simulink model "sm_SG"  (R2019a)
settings: Solver=FixedStepDiscrete  StartTime=0.0  StopTime=stop_time  RelTol=1e-3
InitFcn:
  | sm_callback_init
StopFcn:
  | sm_callback_stop
values from neighbouring files (symbols this model uses):
  mp = sm_init_avalon_signals(mp)    [sm_callback_init.m]
libraries: simulink x3
settings Model: Creator=Ross  LastModifiedBy=Ross
settings DataIOCC: ReturnWorkspaceOutputs=off
settings OptimizationCC: BlockReduction=off  ConditionallyExecuteInputs=off  DefaultParameterBehavior=Inlined
settings DebuggingCC: ReadBeforeWriteMsg=DisableAll  WriteAfterWriteMsg=DisableAll  WriteAfterReadMsg=DisableAll  AlgebraicLoopMsg=error  MultiTaskDSMMsg=none  SingleTaskRateTransMsg=error  PregeneratedLibrarySubsystemCodeDiagnostic=none  ArithmeticOperatorsInVariantConditions=warning
settings HardwareCC: ProdBitPerPointer=32  ProdBitPerSizeT=32  ProdBitPerPtrDiffT=32  ProdLargestAtomicFloat=None  ProdIntDivRoundTo=Undefined  ProdEndianess=Unspecified  ProdWordSize=32  ProdHWDeviceType=ASIC/FPGA->ASIC/FPGA  TargetBitPerPointer=64  TargetBitPerSizeT=64  TargetBitPerPtrDiffT=64  TargetLongLongMode=on  TargetIntDivRoundTo=Zero  TargetEndianess=LittleEndian  TargetWordSize=64  TargetHWDeviceType=Custom Processor->MATLAB Host Computer  ProdEqTarget=off
settings ModelReferenceCC: UpdateModelReferenceTargets=IfOutOfDate
settings SFSimCC: SFSimEcho=off  SimUseLocalCustomCode=off
settings RTWCC: RTWUseLocalCustomCode=off

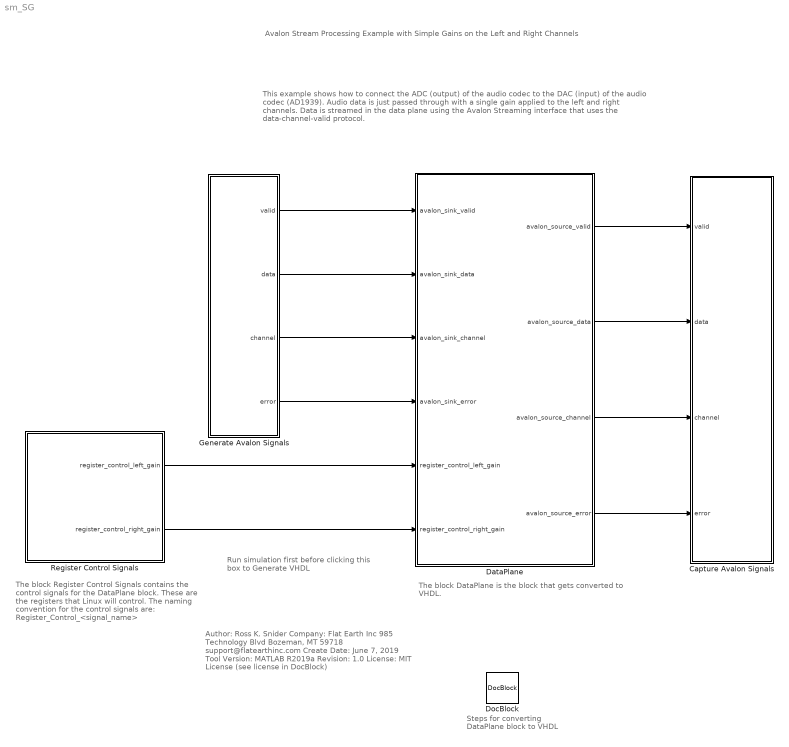
== system sm_SG ==
  note: The block DataPlane is the block that gets converted to VHDL.
  note: Author:          Ross K. Snider
      | Company:     Flat Earth Inc
      |                       985 Technology Blvd
      |                       Bozeman, MT 59718
      |                       support@flatearthinc.com
      | Create Date:  June 7, 2019
      | Tool Version:  MATLAB R2019a
      | Revision:        1.0
      | License:          MIT License (see license in DocBlock)
  note: This example shows how to connect the ADC (output) of the audio codec to the DAC (input) of the audio codec (AD1939). Audio data is just passed through with a single gain applied to the left and right channels. Data is streamed in the data plane using the Avalon Streaming interface that uses the data-channel-valid protocol.
  note: Steps for converting
      | DataPlane block
      | to VHDL
  note: Avalon Stream Processing Example
      | with Simple Gains on the Left and Right Channels
  note: Run simulation first
      | before clicking this box to
      | Generate VHDL
  note: The block Register Control Signals contains
      | the control signals for the DataPlane block.
      | These are the registers that Linux will control.
      | The naming convention for the control
      | signals are:  Register_Control_<signal_name>
  Capture Avalon Signals : Subsystem
  DataPlane : Subsystem  TreatAsAtomicUnit=on
  DocBlock : simulink/Model-Wide Utilities/DocBlock  DocumentType=HTML
  Generate Avalon Signals : Subsystem
  Register Control Signals : Subsystem
  wires:
  Generate Avalon Signals/2(data) -> DataPlane/2(avalon_sink_data)
  Generate Avalon Signals/1(valid) -> DataPlane/1(avalon_sink_valid)
  Generate Avalon Signals/3(channel) -> DataPlane/3(avalon_sink_channel)
  Generate Avalon Signals/4(error) -> DataPlane/4(avalon_sink_error)
  DataPlane/2(avalon_source_data) -> Capture Avalon Signals/2(data)
  DataPlane/1(avalon_source_valid) -> Capture Avalon Signals/1(valid)
  DataPlane/3(avalon_source_channel) -> Capture Avalon Signals/3(channel)
  DataPlane/4(avalon_source_error) -> Capture Avalon Signals/4(error)
  Register Control Signals/1(register_control_left_gain) -> DataPlane/5(register_control_left_gain)
  Register Control Signals/2(register_control_right_gain) -> DataPlane/6(register_control_right_gain)

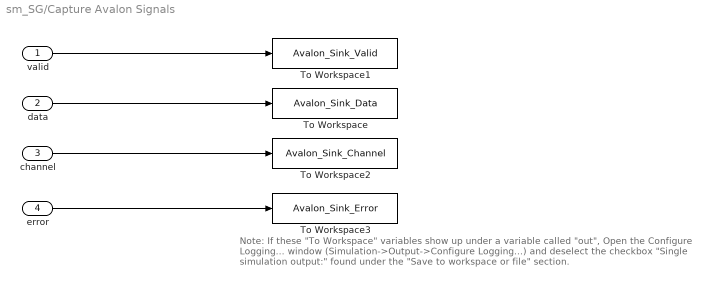
== system sm_SG/Capture Avalon Signals ==
  note: Note:  If these "To Workspace" variables show up under a variable called "out",
      | Open the Configure Logging... window (Simulation->Output->Configure Logging...)
      | and deselect the checkbox "Single simulation output:" found under the "Save to workspace or file" section.
  valid : Inport
  data : Inport  Port=2
  channel : Inport  Port=3
  error : Inport  Port=4
  To Workspace : ToWorkspace  VariableName=Avalon_Sink_Data  SaveFormat=Timeseries  SampleTime=-1
  To Workspace1 : ToWorkspace  VariableName=Avalon_Sink_Valid  SaveFormat=Timeseries  SampleTime=-1
  To Workspace2 : ToWorkspace  VariableName=Avalon_Sink_Channel  SaveFormat=Timeseries  SampleTime=-1
  To Workspace3 : ToWorkspace  VariableName=Avalon_Sink_Error  SaveFormat=Timeseries  SampleTime=-1
  wires:
  data/1 -> To Workspace/1
  valid/1 -> To Workspace1/1
  error/1 -> To Workspace3/1
  channel/1 -> To Workspace2/1

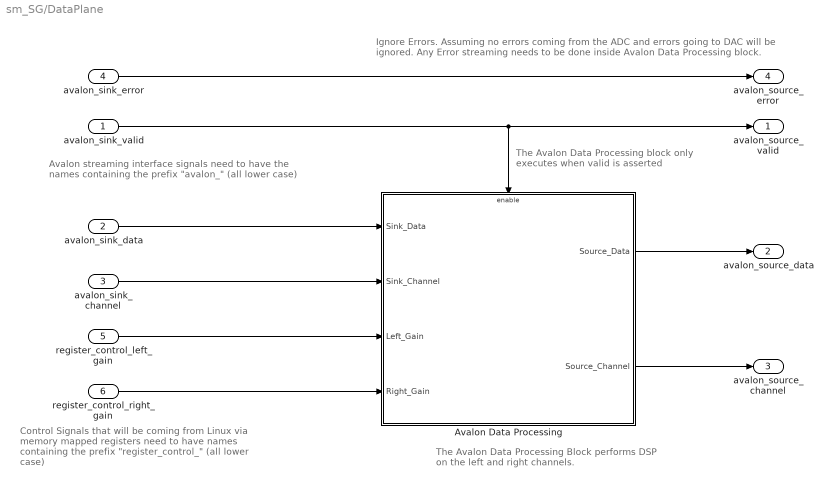
== system sm_SG/DataPlane ==
  note: Control Signals that will be coming from Linux via
      | memory mapped registers need to have names
      | containing the prefix "register_control_"
      | (all lower case)
  note: The Avalon Data Processing Block
      | performs DSP on the left and right channels.
  note: The Avalon Data Processing block
      | only executes when valid is asserted
  note: Ignore Errors.
      | Assuming no errors coming from the ADC and errors going to DAC will be ignored.
      | Any Error streaming needs to be done inside Avalon Data Processing block.
  note: Avalon streaming interface signals need to have the
      | names containing the prefix "avalon_"
      | (all lower case)
  avalon_sink_valid : Inport
  avalon_sink_data : Inport  Port=2
  avalon_sink_channel : Inport  Port=3
  avalon_sink_error : Inport  Port=4
  register_control_left_gain : Inport  Port=5
  register_control_right_gain : Inport  Port=6
  Avalon Data Processing : Subsystem  TreatAsAtomicUnit=on
  avalon_source_valid : Outport
  avalon_source_data : Outport  Port=2
  avalon_source_channel : Outport  Port=3
  avalon_source_error : Outport  Port=4
  wires:
  avalon_sink_channel/1 -> Avalon Data Processing/2(Sink_Channel)
  avalon_sink_error/1 -> avalon_source_error/1
  Avalon Data Processing/1(Source_Data) -> avalon_source_data/1
  avalon_sink_valid/1 -> avalon_source_valid/1, Avalon Data Processing/Enable
  avalon_sink_data/1 -> Avalon Data Processing/1(Sink_Data)
  Avalon Data Processing/2(Source_Channel) -> avalon_source_channel/1
  register_control_right_gain/1 -> Avalon Data Processing/4(Right_Gain)
  register_control_left_gain/1 -> Avalon Data Processing/3(Left_Gain)

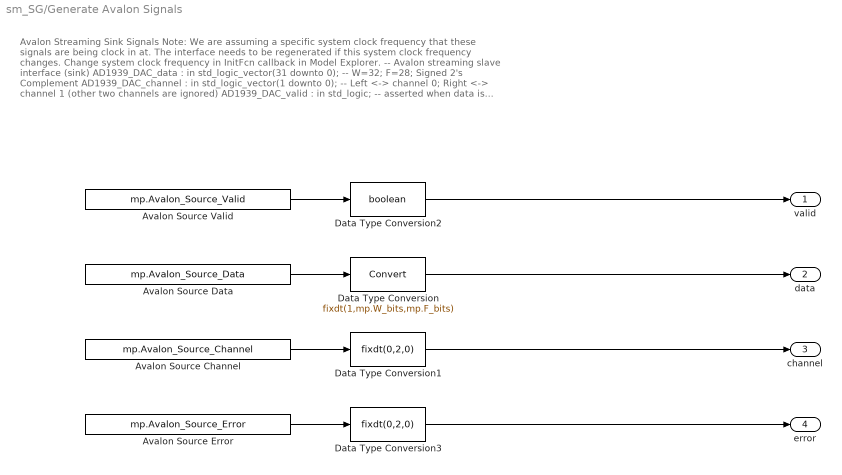
== system sm_SG/Generate Avalon Signals ==
  note: Avalon Streaming Sink Signals
      | Note: We are assuming a specific system clock frequency that these signals are being clock in at.
      | The interface needs to be regenerated if this system clock frequency changes. Change system clock frequency in InitFcn callback in Model Explorer.
      |
      | -- Avalon streaming slave interface (sink)
      | AD1939_DAC_data : in std_logic_vector(31 downto 0); -- W=32; F=28; Signed 2's Complement
      | AD1939_DAC_channel : in std_logic_vector(1 downto 0); -- Left <-> channel 0; Right <-> channel 1 (other two channels are ignored)
      | AD1939_DAC_valid : in std_logic; -- asserted when data is valid
      | AD1939_DAC_error : in std_logic_vector(1 downto 0) -- error channel is ignored, assumed to be error free at this point
      |
      | For more information on the data-channel-valid protocol, s ee chapter 5 in Intel's Avalon Interfaced Specification (p. 40) at https://www.intel.com/content/dam/www/programmable/us/en/pdfs/literature/manual/mnl_avalon_spec.pdf
  Avalon Source Channel : FromWorkspace  VariableName=mp.Avalon_Source_Channel  OutDataTypeStr=double  SampleTime=mp.Ts_system
  "Avalon Source Data " : FromWorkspace  VariableName=mp.Avalon_Source_Data  OutDataTypeStr=double  SampleTime=mp.Ts_system
  Avalon Source Error : FromWorkspace  VariableName=mp.Avalon_Source_Error  OutDataTypeStr=double  SampleTime=mp.Ts_system
  Avalon Source Valid : FromWorkspace  VariableName=mp.Avalon_Source_Valid  OutDataTypeStr=double  SampleTime=mp.Ts_system
  Data Type Conversion : DataTypeConversion  OutDataTypeStr=fixdt(1,mp.W_bits,mp.F_bits)
  Data Type Conversion1 : DataTypeConversion  OutDataTypeStr=fixdt(0,2,0)
  Data Type Conversion2 : DataTypeConversion  OutDataTypeStr=boolean
  Data Type Conversion3 : DataTypeConversion  OutDataTypeStr=fixdt(0,2,0)
  valid : Outport
  data : Outport  Port=2
  channel : Outport  Port=3
  error : Outport  Port=4
  wires:
  Data Type Conversion1/1 -> channel/1
  Data Type Conversion2/1 -> valid/1
  Avalon Source Error/1 -> Data Type Conversion3/1
  Data Type Conversion/1 -> data/1
  Avalon Source Valid/1 -> Data Type Conversion2/1
  Data Type Conversion3/1 -> error/1
  Avalon Source Channel/1 -> Data Type Conversion1/1
  "Avalon Source Data "/1 -> Data Type Conversion/1

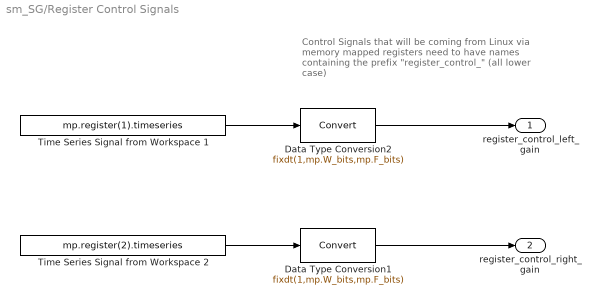
== system sm_SG/Register Control Signals ==
  note: Control Signals that will be coming from Linux via
      | memory mapped registers need to have names
      | containing the prefix "register_control_"
      | (all lower case)
  Data Type Conversion1 : DataTypeConversion  OutDataTypeStr=fixdt(1,mp.W_bits,mp.F_bits)
  Data Type Conversion2 : DataTypeConversion  OutDataTypeStr=fixdt(1,mp.W_bits,mp.F_bits)
  Time Series Signal from Workspace 1 : FromWorkspace  VariableName=mp.register(1).timeseries  OutDataTypeStr=double  SampleTime=mp.Ts_system
  Time Series Signal from Workspace 2 : FromWorkspace  VariableName=mp.register(2).timeseries  OutDataTypeStr=double  SampleTime=mp.Ts_system
  register_control_left_gain : Outport
  register_control_right_gain : Outport  Port=2
  wires:
  Time Series Signal from Workspace 1/1 -> Data Type Conversion2/1
  Time Series Signal from Workspace 2/1 -> Data Type Conversion1/1
  Data Type Conversion2/1 -> register_control_left_gain/1
  Data Type Conversion1/1 -> register_control_right_gain/1

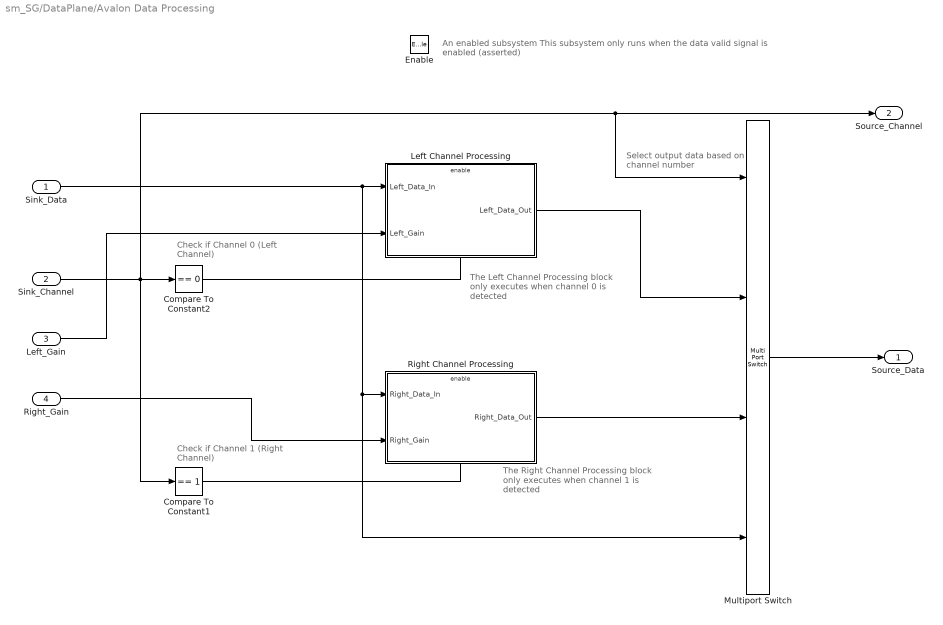
== system sm_SG/DataPlane/Avalon Data Processing ==
  note: Select output data
      | based on channel number
  note: Check if Channel 0
      | (Left Channel)
  note: The Left Channel Processing block
      | only executes when channel 0
      | is detected
  note: The Right Channel Processing block
      | only executes when channel 1
      | is detected
  note: Check if Channel 1
      | (Right Channel)
  note: An enabled subsystem
      | This subsystem only runs when the data valid signal is enabled (asserted)
  Sink_Data : Inport
  Sink_Channel : Inport  Port=2
  Left_Gain : Inport  Port=3
  Right_Gain : Inport  Port=4
  Enable : EnablePort
  Compare To Constant1 : simulink/Logic and Bit Operations/Compare To Constant  relop===  const=1  OutDataTypeStr=boolean
  Compare To Constant2 : simulink/Logic and Bit Operations/Compare To Constant  relop===  const=0  OutDataTypeStr=boolean
  Left Channel Processing : Subsystem  TreatAsAtomicUnit=on
  Multiport Switch : MultiPortSwitch  DataPortOrder=Zero-based contiguous  zeroidx=on
  Right Channel Processing : Subsystem  TreatAsAtomicUnit=on
  Source_Data : Outport  InitialOutput=0
  Source_Channel : Outport  Port=2  InitialOutput=0
  wires:
  Sink_Channel/1 -> Source_Channel/1, Multiport Switch/1, Compare To Constant1/1, Compare To Constant2/1
  Compare To Constant2/1 -> Left Channel Processing/Enable
  Compare To Constant1/1 -> Right Channel Processing/Enable
  Sink_Data/1 -> Multiport Switch/4, Right Channel Processing/1(Right_Data_In), Left Channel Processing/1(Left_Data_In)
  Left Channel Processing/1("Left_Data_Out ") -> Multiport Switch/2
  Right Channel Processing/1("Right_Data_Out ") -> Multiport Switch/3
  Multiport Switch/1 -> Source_Data/1
  Left_Gain/1 -> Left Channel Processing/2(Left_Gain)
  Right_Gain/1 -> Right Channel Processing/2(Right_Gain)

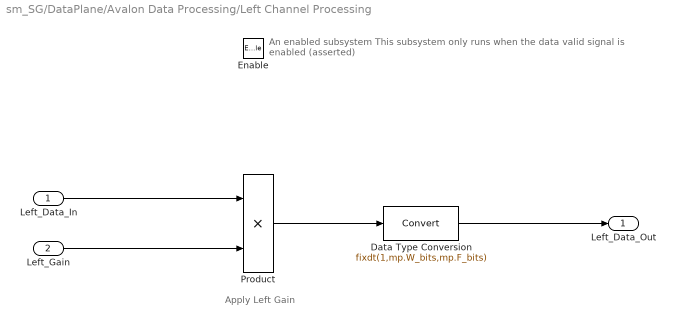
== system sm_SG/DataPlane/Avalon Data Processing/Left Channel Processing ==
  note: Apply Left Gain
  note: An enabled subsystem
      | This subsystem only runs when the data valid signal is enabled (asserted)
  Left_Data_In : Inport
  Left_Gain : Inport  Port=2
  Enable : EnablePort
  Data Type Conversion : DataTypeConversion  OutDataTypeStr=fixdt(1,mp.W_bits,mp.F_bits)
  Product : Product
  "Left_Data_Out " : Outport  InitialOutput=0
  wires:
  Left_Data_In/1 -> Product/1
  Product/1 -> Data Type Conversion/1
  Data Type Conversion/1 -> "Left_Data_Out "/1
  Left_Gain/1 -> Product/2

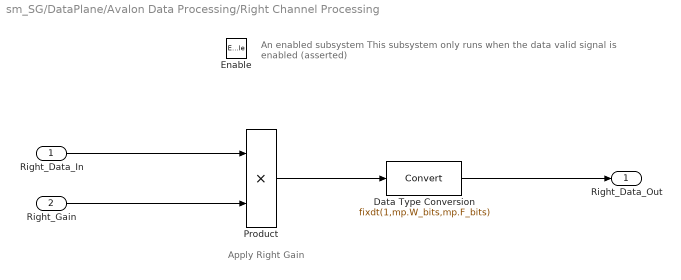
== system sm_SG/DataPlane/Avalon Data Processing/Right Channel Processing ==
  note: Apply Right Gain
  note: An enabled subsystem
      | This subsystem only runs when the data valid signal is enabled (asserted)
  Right_Data_In : Inport
  Right_Gain : Inport  Port=2
  Enable : EnablePort
  Data Type Conversion : DataTypeConversion  OutDataTypeStr=fixdt(1,mp.W_bits,mp.F_bits)
  Product : Product
  "Right_Data_Out " : Outport  InitialOutput=0
  wires:
  Data Type Conversion/1 -> "Right_Data_Out "/1
  Product/1 -> Data Type Conversion/1
  Right_Data_In/1 -> Product/1
  Right_Gain/1 -> Product/2
